simulink model "Example_3Stage"  (Simulink 8.3)
settings: Solver=FixedStepDiscrete  StartTime=0.0  StopTime=1  FixedStep=1  RelTol=1e-3
libraries: CaffeLibrary x13
settings Model: Creator=gipadmin  LastModifiedBy=gipadmin
settings DataIOCC: SignalLoggingSaveFormat=Dataset
settings DebuggingCC: UnderspecifiedInitializationDetection=Simplified  StateNameClashWarn=none
settings GRTTargetCC: CombineOutputUpdateFcns=on  GRTInterface=off

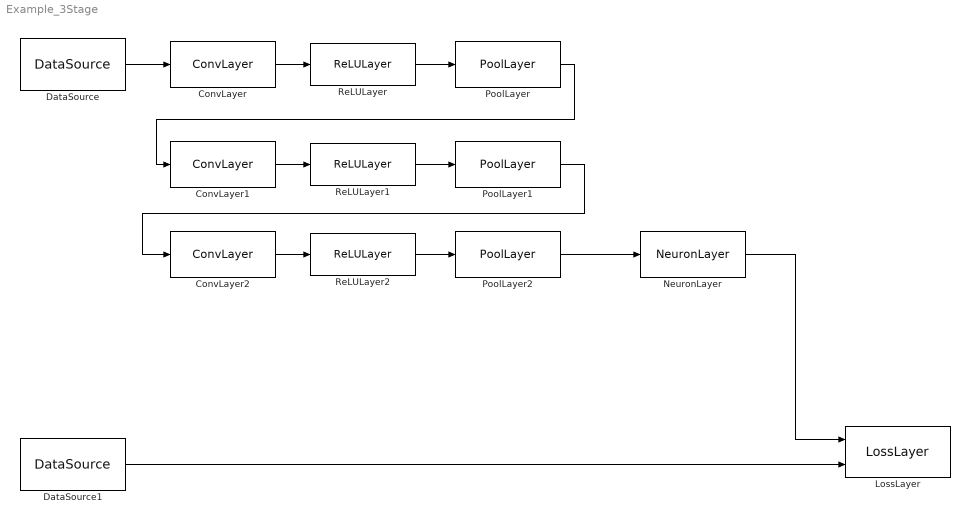
== system Example_3Stage ==
  ConvLayer : CaffeLibrary/ConvLayer  title=0  numFilters=24.759999999999998  kernelSize=1.0  stride=0  weightFill=Xavier  weightStd=0  biasFill=0  biasVal=0
  ConvLayer1 : CaffeLibrary/ConvLayer  title=0  numFilters=24.759999999999998  kernelSize=1.0  stride=0  weightFill=Xavier  weightStd=0  biasFill=0  biasVal=0
  ConvLayer2 : CaffeLibrary/ConvLayer  title=0  numFilters=24.759999999999998  kernelSize=1.0  stride=0  weightFill=Xavier  weightStd=0  biasFill=0  biasVal=0
  DataSource : CaffeLibrary/DataSource  title=HDF5  srcFile=file.txt  batchSize=58
  DataSource1 : CaffeLibrary/DataSource  title=HDF5  srcFile=file.txt  batchSize=58
  LossLayer : CaffeLibrary/LossLayer  title=EuclideanLoss
  NeuronLayer : CaffeLibrary/NeuronLayer  title=Neuron  typeOf=Sigmoid
  PoolLayer : CaffeLibrary/PoolLayer  title=Pooling  poolType=MAX  kernelSize=1.000  stride=0.0
  PoolLayer1 : CaffeLibrary/PoolLayer  title=Pooling  poolType=MAX  kernelSize=1.000  stride=0.0
  PoolLayer2 : CaffeLibrary/PoolLayer  title=Pooling  poolType=MAX  kernelSize=1.000  stride=0.0
  ReLULayer : CaffeLibrary/ReLULayer
  ReLULayer1 : CaffeLibrary/ReLULayer
  ReLULayer2 : CaffeLibrary/ReLULayer
  wires:
  DataSource/1 -> ConvLayer/1
  ConvLayer/1 -> ReLULayer/1
  ReLULayer/1 -> PoolLayer/1
  PoolLayer/1 -> ConvLayer1/1
  ConvLayer1/1 -> ReLULayer1/1
  ReLULayer1/1 -> PoolLayer1/1
  PoolLayer1/1 -> ConvLayer2/1
  ConvLayer2/1 -> ReLULayer2/1
  ReLULayer2/1 -> PoolLayer2/1
  PoolLayer2/1 -> NeuronLayer/1
  NeuronLayer/1 -> LossLayer/1
  DataSource1/1 -> LossLayer/2
